simulink model "uz_approximate_flux_d"  (R2023b)
settings: Solver=FixedStepDiscrete  StartTime=0.0  StopTime=0.1  RelTol=1e-3  EnableMultiTasking=on
PreLoadFcn:
  | uz_setCodegenPaths
model workspace (MATLAB code in the model file):
  | cmdLim = Simulink.Parameter;
  | cmdLim.Value = 15;
  | cmdLim.Description = 'Limit for controlling the maximum surface command angle.';
  | cmdLim.Min = 0;
  | cmdLim.Max = 90;
  | cmdLim.DocUnits = 'deg';
  | 
  | dispGain = Simulink.Parameter;
  | dispGain.Value = 0.75;
  | dispGain.Description = 'Gain applied to the displacement error.';
  | dispGain.Min = 0;
  | dispGain.Max = [];
  | dispGain.DocUnits = 'deg/sec/deg';
  | 
  | dispLim = Simulink.Parameter;
  | dispLim.Value = 30;
  | dispLim.Description = 'Limit for controlling the maximum commanded angle.';
  | dispLim.Min = 0;
  | dispLim.Max = 180;
  | dispLim.DocUnits = 'deg';
  | 
  | intGain = Simulink.Parameter;
  | intGain.Value = 0.5;
  | intGain.Description = 'Gain applied to the integral error.';
  | intGain.Min = 0;
  | intGain.Max = [];
  | intGain.DocUnits = 'deg/sec/deg/sec';
  | 
  | intLim = Simulink.Parameter;
  | intLim.Value = 5;
  | intLim.Description = 'Limit for controlling the maximum commanded angle.';
  | intLim.Min = 0;
  | intLim.Max = 90;
  | intLim.DocUnits = 'deg';
  | 
  | rateGain = Simulink.Parameter;
  | rateGain.Value = 2;
  | rateGain.Description = 'Gain applied to the rate error.';
  | rateGain.Min = 0;
  | rateGain.Max = [];
  | rateGain.DocUnits = 'deg/deg/sec';
  | 
  | rateLim = Simulink.Parameter;
  | rateLim.Value = 6;
  | rateLim.Description = 'Limit for controlling the maximum commanded angle.';
  | rateLim.Min = 0;
  | rateLim.Max = 180;
  | rateLim.DocUnits = 'deg/sec';
  | 
  | hdgGain = Simulink.Parameter;
  | hdgGain.Value = 0.015;
settings Model: RequirementInfo={} %GIDa_fe9045fd_0412_4b6e_8206_617cc20e6fde  FPTRunName=Active  Creator=ts  LastModifiedBy=Philipp
settings SolverCC: AlgebraicLoopSolver=TrustRegion  PositivePriorityOrder=on  AutoInsertRateTranBlk=on
settings DataIOCC: SaveOutput=off  SignalLogging=off  DSMLogging=off  SaveTime=off
settings OptimizationCC: DefaultParameterBehavior=Inlined  UseDivisionForNetSlopeComputation=on  GainParamInheritBuiltInType=on  UseFloatMulNetSlope=on  UseSpecifiedMinMax=on  InlineInvariantSignals=on  PassReuseOutputArgsAs=Individual arguments  NoFixptDivByZeroProtection=on  EfficientFloat2IntCast=on  LifeSpan=1  MaxStackSize=64  OptimizeBlockOrder=speed  DifferentSizesBufferReuse=on  EfficientTunableParamExpr=on
settings DebuggingCC: UnconnectedInputMsg=warning  UnconnectedOutputMsg=warning  UnconnectedLineMsg=warning  AllowSymbolicDim=off  SFUnexpectedBacktrackingDiag=warning  SFNoUnconditionalDefaultTransitionDiag=warning  SFExecutionAtInitializationDiag=none  ArithmeticOperatorsInVariantConditions=warning
settings HardwareCC: ProdBitPerPointer=32  ProdBitPerSizeT=32  ProdBitPerPtrDiffT=32  ProdLargestAtomicInteger=Long  ProdLargestAtomicFloat=Double  ProdWordSize=32  ProdLongLongMode=on  ProdHWDeviceType=ARM Compatible->ARM Cortex-R  HardwareBoardFeatureSet=SoCBlockset
settings ModelReferenceCC: EnableRefExpFcnMdlSchedulingChecks=on
settings SFSimCC: MATLABDynamicMemAlloc=off
settings RTWCC: Description=Embedded Coder  SystemTargetFile=ert.tlc  GenCodeOnly=on  TemplateMakefile=ert_default_tmf  GenerateReport=on  BuildConfiguration=Faster Runs  IncludeHyperlinkInReport=on  GenerateCodeMetricsReport=on  CheckMdlBeforeBuild=Warning  DLArmComputeVersion=19.05
settings CodeAppCC: ForceParamTrailComments=on  IgnoreCustomStorageClasses=off  OperatorAnnotations=on  SimulinkDataObjDesc=on  SFDataObjDesc=on  MATLABFcnDesc=on  CustomSymbolStrGlobalVar=rt$N$M  CustomSymbolStrType=$N$M  CustomSymbolStrFcn=$N$M$F  CustomSymbolStrMacro=$N$M  InsertBlockDesc=on  StateflowObjectComments=on  MATLABSourceComments=on  EnableCustomComments=on  ReqsInCode=on
settings ERTTargetCC: TargetLangStandard=C99 (ISO)  CodeReplacementLibrary=GNU C99 extensions  MultiwordLength=2048  IncludeMdlTerminateFcn=off  CombineSignalStateStructs=on  SuppressErrorStatus=on  IncludeFileDelimiter=UseQuote  SupportAbsoluteTime=off  CodeInterfacePackaging=Reusable function  SupportNonFinite=off  RemoveResetFunc=off  InlinedParameterPlacement=NonHierarchical  MultiInstanceErrorCode=Warning  RootIOFormat=Part of model data structure  ERTCustomFileTemplate=example_file_process.tlc  GlobalDataDefinition=InSourceFile  GlobalDataReference=InSourceFile  ERTFilePackagingFormat=CompactWithDataFile
settings ConfigComp: CovScope=ReferencedModels  CovSaveName=covdata_rollAP  CovMetricSettings=dcmtrwe  CovHTMLOptions=-sRT=1 -aTS=1 -bRG=1 -bTC=1 -hTR=1 -nFC=0 -scm=1 -bcm=1 -xEv=0  CovSaveCumulativeToWorkspaceVar=on  CovSaveSingleToWorkspaceVar=on  CovCumulativeVarName=covCumulativeData_rollAP  CovReportOnPause=off  CovExternalEMLEnable=off  CovSFcnEnable=off

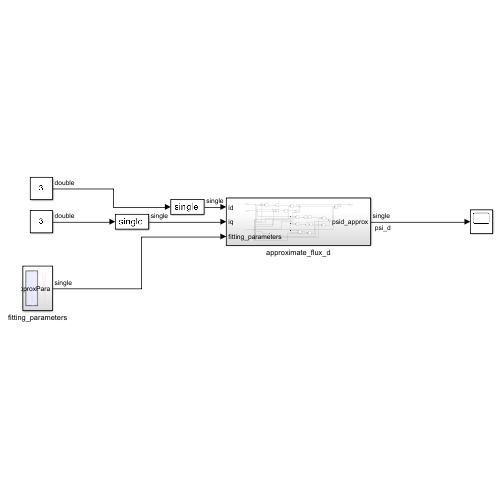
[thumbnail: Simulink's stored preview of the top-level diagram]
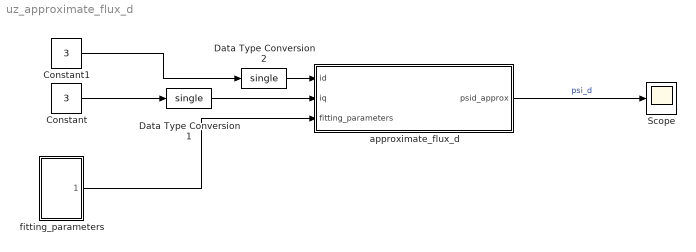
== system uz_approximate_flux_d ==
  Constant : Constant  Value=3
  Constant1 : Constant  Value=3
  Data Type Conversion1 : DataTypeConversion  OutDataTypeStr=single  SaturateOnIntegerOverflow=off  RndMeth=Floor
  Data Type Conversion2 : DataTypeConversion  OutDataTypeStr=single  SaturateOnIntegerOverflow=off  RndMeth=Floor
  Scope : Scope
  approximate_flux_d : Subsystem
  fitting_parameters : Subsystem
  wires:
  approximate_flux_d/1(psid_approx) -> Scope/1  "psi_d"
  fitting_parameters/1(ApproxPara) -> approximate_flux_d/3(fitting_parameters)
  Constant/1 -> Data Type Conversion1/1
  Data Type Conversion1/1 -> approximate_flux_d/2(iq)
  Constant1/1 -> Data Type Conversion2/1
  Data Type Conversion2/1 -> approximate_flux_d/1(id)

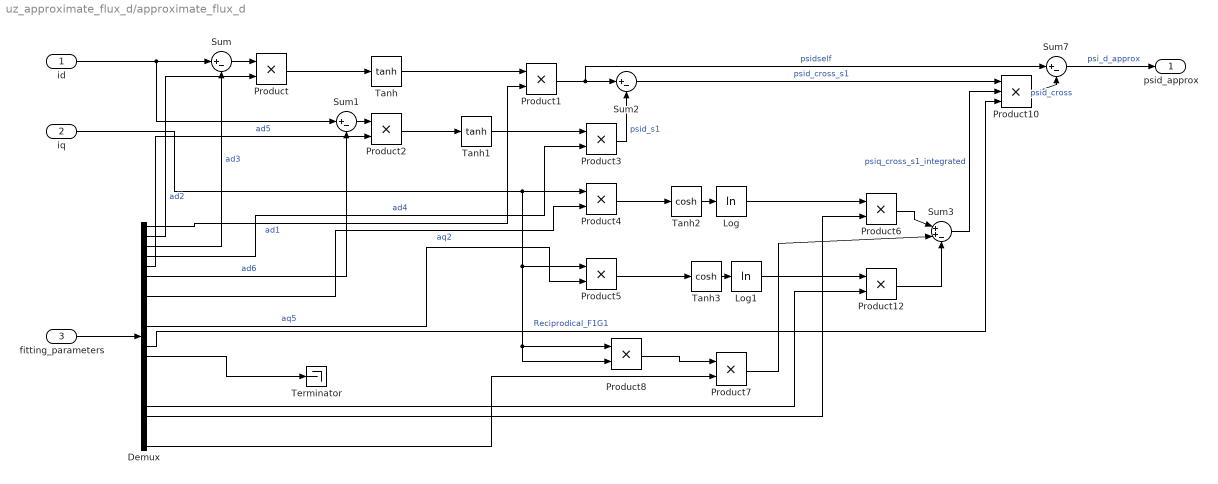
== system uz_approximate_flux_d/approximate_flux_d ==
  id : Inport
  iq : Inport  Port=2
  fitting_parameters : Inport  Port=3
  Demux : Demux  Outputs=23
  Log : Math  Operator=log  SignedPower=on
  Log1 : Math  Operator=log  SignedPower=on
  Product{,1..2,4..5,8} (6 alike) : Product  OutDataTypeStr=Inherit: Same as first input
  Product10 : Product  Inputs=3
  Product{3,6..7,12} (4 alike) : Product
  Sum : Sum  Inputs=|+-  OutDataTypeStr=Inherit: Same as first input
  Sum1 : Sum  Inputs=|+-
  Sum2 : Sum  Inputs=|+-  OutDataTypeStr=Inherit: Same as first input
  Sum3 : Sum  Inputs=|++-  OutDataTypeStr=Inherit: Same as first input
  Sum7 : Sum  Inputs=|+-  OutDataTypeStr=Inherit: Same as first input
  Tanh : Trigonometry  Operator=tanh
  Tanh1 : Trigonometry  Operator=tanh
  Tanh2 : Trigonometry  Operator=cosh
  Tanh3 : Trigonometry  Operator=cosh
  Terminator : Terminator
  psid_approx : Outport
  wires:
  fitting_parameters/1 -> Demux/1
  Demux/1 -> Product1/2  "ad1"
  Demux/3 -> Sum/2  "ad3"
  Sum/1 -> Product/1
  Demux/2 -> Product/2  "ad2"
  Product1/1 -> Sum7/1, Sum2/1  "psidself"
  Demux/4 -> Product3/2  "ad4"
  Sum1/1 -> Product2/1
  Demux/5 -> Product2/2  "ad5"
  Demux/6 -> Sum1/2  "ad6"
  id/1 -> Sum1/1, Sum/1
  Product3/1 -> Sum2/2  "psid_s1"
  iq/1 -> Product8/2, Product8/1, Product5/1, Product4/1
  Sum2/1 -> Product10/1  "psid_cross_s1"
  Tanh2/1 -> Log/1
  Tanh3/1 -> Log1/1
  Product8/1 -> Product7/1
  Product7/1 -> Sum3/2
  Demux/20 -> Product6/2
  Product6/1 -> Sum3/1
  Demux/19 -> Product12/2
  Product12/1 -> Sum3/3
  Sum3/1 -> Product10/2  "psiq_cross_s1_integrated"
  Demux/11 -> Product5/2  "aq5"
  Demux/8 -> Product4/2  "aq2"
  Product10/1 -> Sum7/2  "psid_cross"
  Sum7/1 -> psid_approx/1  "psi_d_approx"
  Demux/14 -> Terminator/1
  Demux/13 -> Product10/3  "Reciprodical_F1G1"
  Log/1 -> Product6/1
  Log1/1 -> Product12/1
  Tanh/1 -> Product1/1
  Tanh1/1 -> Product3/1
  Product/1 -> Tanh/1
  Product2/1 -> Tanh1/1
  Product4/1 -> Tanh2/1
  Product5/1 -> Tanh3/1
  Demux/23 -> Product7/2

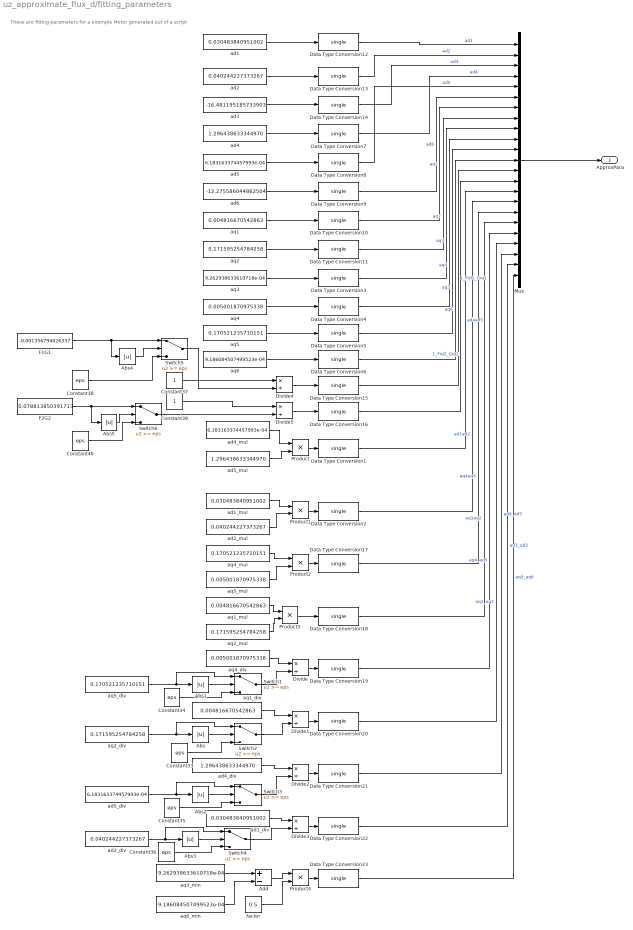
== system uz_approximate_flux_d/fitting_parameters ==
  note: These are fitting parameters for a example Motor generated out of a script
  Abs{,1..5} (6 alike) : Abs  SaturateOnIntegerOverflow=off
  Add : Sum  Inputs=+-
  Constant{33..36,38,40} (6 alike) : Constant  Value=eps
  Constant37 : Constant
  Constant39 : Constant
  Data Type Conversion{1..23} (23 alike) : DataTypeConversion  OutDataTypeStr=single  SaturateOnIntegerOverflow=off  RndMeth=Floor
  Divide{,1..5} (6 alike) : Product  Inputs=*/
  F1G1 : Constant  Value=-0.001356794026337
  F2G2 : Constant  Value=0.078813850391713
  Mux : Mux  Inputs=23
  Product{,1..4} (5 alike) : Product
  Switch{1..6} (6 alike) : Switch  Threshold=eps  SaturateOnIntegerOverflow=off  InputSameDT=off
  ad1 : Constant  Value=0.030483840951002
  ad1_div : Constant  Value=0.030483840951002
  ad1_mul : Constant  Value=0.030483840951002
  ad2 : Constant  Value=0.040244227373267
  ad2_div : Constant  Value=0.040244227373267
  ad2_mul : Constant  Value=0.040244227373267
  ad3 : Constant  Value=-16.481195185733903
  ad4 : Constant  Value=1.296438633344970
  ad4_div : Constant  Value=1.296438633344970
  ad4_mul : Constant  Value=6.183163374457993e-04
  ad5 : Constant  Value=6.183163374457993e-04
  ad5_div : Constant  Value=6.183163374457993e-04
  ad5_mul : Constant  Value=1.296438633344970
  ad6 : Constant  Value=-12.275586044862504
  aq1 : Constant  Value=0.004816670542863
  aq1_div : Constant  Value=0.004816670542863
  aq1_mul : Constant  Value=0.004816670542863
  aq2 : Constant  Value=0.171595254784258
  aq2_div : Constant  Value=0.171595254784258
  aq2_mul : Constant  Value=0.171595254784258
  aq3 : Constant  Value=9.262938633610718e-04
  aq3_min : Constant  Value=9.262938633610718e-04
  aq4 : Constant  Value=0.005001870975338
  aq4_div : Constant  Value=0.005001870975338
  aq4_mul : Constant  Value=0.170521235710151
  aq5 : Constant  Value=0.170521235710151
  aq5_div : Constant  Value=0.170521235710151
  aq5_mul : Constant  Value=0.005001870975338
  aq6 : Constant  Value=9.186084507499523e-04
  aq6_min : Constant  Value=9.186084507499523e-04
  factor : Constant  Value=0.5  OutDataTypeStr=double  SampleTime=-1
  ApproxPara : Outport
  wires:
  ad1/1 -> Data Type Conversion12/1
  ad4/1 -> Data Type Conversion7/1
  Data Type Conversion14/1 -> Mux/3  "ad3"
  Data Type Conversion11/1 -> Mux/8  "aq2"
  ad3/1 -> Data Type Conversion14/1
  Data Type Conversion9/1 -> Mux/6  "ad6"
  Data Type Conversion12/1 -> Mux/1  "ad1"
  Data Type Conversion10/1 -> Mux/7  "aq1"
  aq2/1 -> Data Type Conversion11/1
  ad6/1 -> Data Type Conversion9/1
  Data Type Conversion13/1 -> Mux/2  "ad2"
  Data Type Conversion7/1 -> Mux/4  "ad4"
  ad5/1 -> Data Type Conversion8/1
  aq1/1 -> Data Type Conversion10/1
  Data Type Conversion8/1 -> Mux/5  "ad5"
  ad2/1 -> Data Type Conversion13/1
  Data Type Conversion3/1 -> Mux/9  "aq3"
  aq3/1 -> Data Type Conversion3/1
  Data Type Conversion4/1 -> Mux/10  "aq4"
  aq4/1 -> Data Type Conversion4/1
  Data Type Conversion5/1 -> Mux/11  "aq5"
  aq5/1 -> Data Type Conversion5/1
  Data Type Conversion6/1 -> Mux/12  "aq6"
  aq6/1 -> Data Type Conversion6/1
  Data Type Conversion15/1 -> Mux/13  "1_Fid1_Giq1"
  Data Type Conversion16/1 -> Mux/14  "1_Fid2_Giq2"
  ad4_mul/1 -> Product/1
  ad5_mul/1 -> Product/2
  Product/1 -> Data Type Conversion1/1
  Data Type Conversion1/1 -> Mux/15  "ad4ad5"
  Data Type Conversion2/1 -> Mux/16  "ad1ad2"
  ad1_mul/1 -> Product1/1
  ad2_mul/1 -> Product1/2
  Product1/1 -> Data Type Conversion2/1
  aq4_mul/1 -> Product2/1
  aq5_mul/1 -> Product2/2
  Product2/1 -> Data Type Conversion17/1
  Data Type Conversion18/1 -> Mux/18  "aq1aq2"
  Product3/1 -> Data Type Conversion18/1
  aq2_mul/1 -> Product3/2
  aq1_mul/1 -> Product3/1
  Data Type Conversion17/1 -> Mux/17  "aq4aq5"
  Divide/1 -> Data Type Conversion19/1
  aq4_div/1 -> Divide/1
  Data Type Conversion19/1 -> Mux/19  "aq4_aq5"
  aq1_div/1 -> Divide1/1
  Data Type Conversion20/1 -> Mux/20  "aq1_aq2"
  Divide1/1 -> Data Type Conversion20/1
  Divide2/1 -> Data Type Conversion21/1
  Data Type Conversion21/1 -> Mux/21  "ad4_ad5"
  ad4_div/1 -> Divide2/1
  ad1_div/1 -> Divide3/1
  Data Type Conversion22/1 -> Mux/22  "ad1_ad2"
  Divide3/1 -> Data Type Conversion22/1
  aq3_min/1 -> Add/1
  aq6_min/1 -> Add/2
  Data Type Conversion23/1 -> Mux/23  "aq3_aq6"
  Product4/1 -> Data Type Conversion23/1
  factor/1 -> Product4/2
  Add/1 -> Product4/1
  Mux/1 -> ApproxPara/1
  aq2_div/1 -> Switch2/1, Abs/1
  Switch2/1 -> Divide1/2
  Abs/1 -> Switch2/2
  Constant33/1 -> Switch2/3
  aq5_div/1 -> Switch1/1, Abs1/1
  Switch1/1 -> Divide/2
  Abs1/1 -> Switch1/2
  Constant34/1 -> Switch1/3
  ad5_div/1 -> Switch3/1, Abs2/1
  Switch3/1 -> Divide2/2
  Abs2/1 -> Switch3/2
  Constant35/1 -> Switch3/3
  ad2_div/1 -> Switch4/1, Abs3/1
  Switch4/1 -> Divide3/2
  Abs3/1 -> Switch4/2
  Constant36/1 -> Switch4/3
  Abs4/1 -> Switch5/2
  Constant38/1 -> Switch5/3
  Divide4/1 -> Data Type Conversion15/1
  Switch5/1 -> Divide4/2
  F1G1/1 -> Abs4/1, Switch5/1
  Constant37/1 -> Divide4/1
  Constant39/1 -> Divide5/1
  F2G2/1 -> Abs5/1, Switch6/1
  Constant40/1 -> Switch6/3
  Abs5/1 -> Switch6/2
  Divide5/1 -> Data Type Conversion16/1
  Switch6/1 -> Divide5/2
